simulink model "Angel_Motor"  (R2018a)
settings: Solver=VariableStepAuto  StartTime=0.0  StopTime=10  RelTol=1e-3
libraries: simulink x1, vrlib x1
settings Model: Creator=Juan  LastModifiedBy=Juan

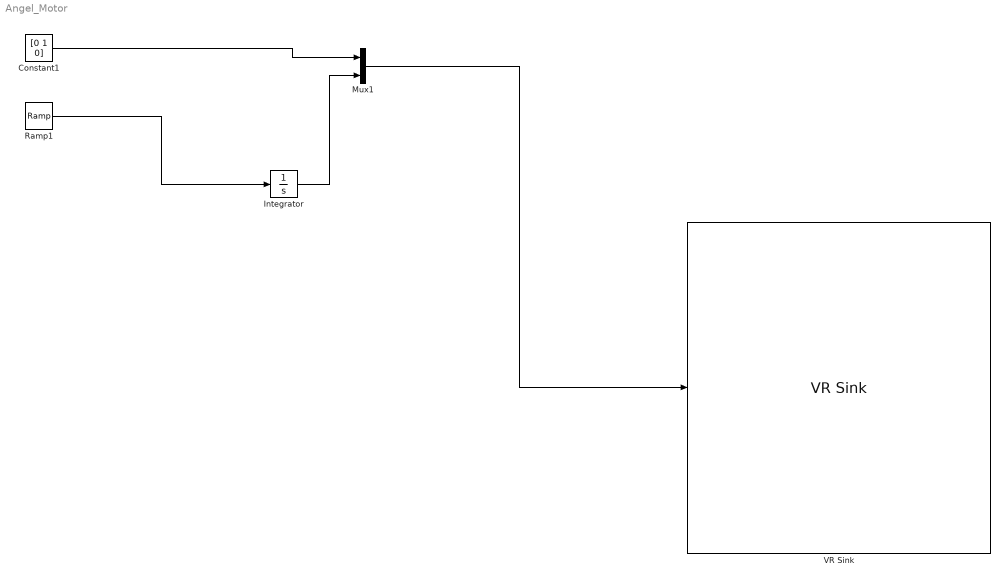
== system Angel_Motor ==
  Constant1 : Constant  Value=[0 1 0]  VectorParams1D=off
  Integrator : Integrator
  Mux1 : Mux  Inputs=2
  Ramp1 : simulink/Sources/Ramp  slope=4  start=0  InitialOutput=0
  VR Sink : vrlib/VR Sink  InstantiateOnLoad=on  SampleTime=0.02  ViewEnable=on  RemoteChange=off  RemoteView=off  FieldsWritten=motor_pin.rotation.4.1.1.double  WorldFileName=F:\MATLAB\EE183DA\Angel_motor.wrl  AutoView=off  VideoDimensions=[]  AllowVariableSize=off  FigureProperties="{'Position', 'Name', 'Viewpoint', 'CameraBound', 'CameraDirection', 'CameraPosition', 'CameraUpVector', 'ZoomFactor', 'Antialiasing', 'Headlight', 'Lighting', 'NavPanel', 'Sound', 'StatusBar', 'Stereo3D', 'Stereo3DCameraOffset', 'Stereo3DHIT', 'ToolBar', 'Textures', 'Transparency', 'Triad', 'Wireframe', 'NavZones', 'NavMode', 'NavSpeed', 'CaptureFileFormat', 'CaptureFileName', 'Record2DCompressMethod', 'Record2DCompressQuality', 'Record2D', 'Record2DFileName', 'Record2DFPS'; [1.3010000000000000e+03   1.7700000000000000e+02   5.7600000000000000e+02   3.5000000000000000e+02], '', '', 'on', [8.7021586712961035e-02   2.1541899679944915e-01  -9.7263657100886580e-01], [-2.3957572147424444e+00   2.7056855110468150e+00   2.6092441370581703e+01], [-4.9892835449784588e-02   9.7605758238612850e-01   2.1171277910728434e-01], [1.0000000000000000e+00], 'on', 'on', 'on', 'halfbar', 'on', 'on', 'off', [1.0000000149011612e-01], [0.0000000000000000e+00], 'on', 'on', 'on', 'none', 'off', 'off', 'fly', 'normal', 'tif', '%f_anim_%n.tif', 'auto', [7.5000000000000000e+01], 'off', '%f_anim_%n.avi', 'auto'}"
      settings: SourceProductBaseCode=VR
  wires:
  Constant1/1 -> Mux1/1
  Mux1/1 -> VR Sink/1
  Ramp1/1 -> Integrator/1
  Integrator/1 -> Mux1/2
